simulink model "Noa_Nofusion_backup"  (R2020b)
settings: Solver=FixedStepDiscrete  StartTime=0.0  StopTime=Inf  FixedStep=0.02  RelTol=1e-3
PostLoadFcn:
  | if any(exist('dsrtsu_mdlpostloadfcn', 'file') ~= 0), dsrtsu_mdlpostloadfcn('Execute', bdroot); end
InitFcn:
  | , if any(exist('rtifpga_mdlclblib', 'file') ~= 0), rtifpga_mdlclblib('Init', bdroot); end,
  | , if any(exist('dsmpb_private', 'file') ~= 0), dsmpb_private('dsmpb_mdlclblib', 'Init', bdroot); end,
undefined symbols (not defined in the file): ACC_TimeGap_DecSetSwt, ACC_TimeGap_IncSetSwt, AccelPedalPosn, AccelPedalPosnVldty, AccelPedlPosnDiagc, AccPedalOverride, ACU_ShiftInProgress, ADAS_Posn_CurLane, AESSwtReq, ALC_SwtReq, BrkPedalSts, CC_ACC_CANCEL_OFFSwt, CC_ACC_CRUISE_OFFSwt, CC_ACC_DecSetSpd_SetSwt, CC_ACC_IncSetSpd_ResuSwt, CC_ACCSwtErr, CharSpd_ms, CSA_NODE, CURRENT_GEAR, CurrentGearValid, DiscIntNeverNeededParam, DrvDoorSts, DrvSBR, DrvTrqReqOvld, ECMACCInterface, ECMRespACC, ELKSwtReq, EngLimpHomeSts, EngSpd, EngState, EngState_PHEV, EngTrqMaxActSpd, EngTrqMinAct, EPS_DrvInpTrqVal_HighReslolution, EPS_FailSts, EPS_LKATorqOvrlDlvd, EPS_LKATorqOvrlDlvdVld, EPS_LKATrqOvlDlvdSts, EPS_SteerMod, EPS_TrqSnsrSts, EQ4_APPINFO, EQ4_LA_ELEM, EQ4_LA_HDR, EQ4_LAP_ELEM, EQ4_LAP_HDR, EQ4_LH_ELEM, EQ4_LH_HDR, EQ4_LRE_ELEM, EQ4_LRE_HDR, ESS_PedSwtReq, ESS_VehSwtReq, FFogLmpSts_F_Pbox, FLWheelDriveDirection, FLWheelSpd, FrntWiprSwtSts, FrntWshrSwtSts, FRWheelDriveDirection, FRWheelSpd, HazardLmpSwtSts, HCU_AccelPedalPosn_Diag ... (+152)
libraries: simulink x117, dsmpblib x30
(part 9 of 11)

== system Noa_Nofusion_backup/Common/Subsystem7/DS/DriverStsConditnJudge/DSOther2Hi1DrowsnsJudge ==
  note: %Note
      | Conditions of drowsns state from other state to High 1 as follow:
      | DMSSts_ACC is 0x02: Active
      | && HeadDetn is 0x01: Yes
      | && DrowsnsLevel_ACC is 0x3: Hi level Drowsiness
      | && DrowsnsQlty_ACC≥85%
      | && During time≥0.5s(adjustable)
  canDMSSts : Inport
  canHeadDetn : Inport  Port=2
  canDrowsnsLevel : Inport  Port=3
  PtDSOther2Hi1Drowsns : Inport  Port=4
  Compare To Constant : simulink/Logic and Bit Operations/Compare To Constant  relop===  const=2  OutDataTypeStr=boolean
  Compare To Constant1 : simulink/Logic and Bit Operations/Compare To Constant  relop===  const=1  OutDataTypeStr=boolean
  Compare To Constant2 : simulink/Logic and Bit Operations/Compare To Constant  relop===  const=3  OutDataTypeStr=boolean
  Data Type Conversion : DataTypeConversion  OutDataTypeStr=single
  Logical Operator : Logic  Inputs=3  AllPortsSameDT=off  OutDataTypeStr=boolean
  Relational Operator : RelationalOperator  OutDataTypeStr=boolean  RndMeth=Simplest
  counter : DiscreteIntegrator  ExternalReset=either  SampleTime=-1  LimitOutput=on  UpperSaturationLimit=10  LowerSaturationLimit=-10  ICPrevOutput=DiscIntNeverNeededParam  ICPrevScaledInput=DiscIntNeverNeededParam
  DSOther2Hi1Drowsns : Outport
  wires:
  counter/1 -> Relational Operator/1
  Relational Operator/1 -> DSOther2Hi1Drowsns/1
  Compare To Constant2/1 -> Logical Operator/3
  Compare To Constant/1 -> Logical Operator/1
  Compare To Constant1/1 -> Logical Operator/2
  canDrowsnsLevel/1 -> Compare To Constant2/1
  canHeadDetn/1 -> Compare To Constant1/1
  canDMSSts/1 -> Compare To Constant/1
  Logical Operator/1 -> Data Type Conversion/1
  PtDSOther2Hi1Drowsns/1 -> Relational Operator/2
  Data Type Conversion/1 -> counter/2, counter/1

== system Noa_Nofusion_backup/Common/Subsystem7/DS/DriverStsConditnJudge/DSOther2Hi2DistractnJudge ==
  note: %Note
      | Conditions of distraction state from other state to High 2 as follow:
      | DMSSts_ACC is 0x02: Active
      | && HeadDetn is 0x01: Yes
      | && DistrctnLevel_ACC is 0x03: Hi level distraction
      | && DistrctnQlty_ACC≥ 85%
      | && During time≥5s(adjustable)
  canDMSSts : Inport
  canHeadDetn : Inport  Port=2
  canDistrctnLevel : Inport  Port=3
  canDistrctnQlty : Inport  Port=4
  PtDSOther2Hi2Distractn : Inport  Port=5
  Compare To Constant : simulink/Logic and Bit Operations/Compare To Constant  relop===  const=2  OutDataTypeStr=boolean
  Compare To Constant1 : simulink/Logic and Bit Operations/Compare To Constant  relop===  const=1  OutDataTypeStr=boolean
  Compare To Constant2 : simulink/Logic and Bit Operations/Compare To Constant  relop===  const=3  OutDataTypeStr=boolean
  Compare To Constant4 : simulink/Logic and Bit Operations/Compare To Constant  relop=>=  const=85  OutDataTypeStr=boolean
  Compare To Constant8 : simulink/Logic and Bit Operations/Compare To Constant  relop=<=  const=100  OutDataTypeStr=boolean
  Data Type Conversion : DataTypeConversion  OutDataTypeStr=single
  Logical Operator : Logic  Inputs=5  AllPortsSameDT=off  OutDataTypeStr=boolean
  Relational Operator : RelationalOperator  OutDataTypeStr=boolean  RndMeth=Simplest
  counter : DiscreteIntegrator  ExternalReset=either  SampleTime=-1  LimitOutput=on  UpperSaturationLimit=10  LowerSaturationLimit=-10  ICPrevOutput=DiscIntNeverNeededParam  ICPrevScaledInput=DiscIntNeverNeededParam
  DSOther2Hi2Distractn : Outport
  wires:
  counter/1 -> Relational Operator/1
  Relational Operator/1 -> DSOther2Hi2Distractn/1
  Compare To Constant8/1 -> Logical Operator/5
  Compare To Constant4/1 -> Logical Operator/4
  Compare To Constant2/1 -> Logical Operator/3
  Compare To Constant/1 -> Logical Operator/1
  Compare To Constant1/1 -> Logical Operator/2
  canDistrctnQlty/1 -> Compare To Constant4/1, Compare To Constant8/1
  canDistrctnLevel/1 -> Compare To Constant2/1
  canHeadDetn/1 -> Compare To Constant1/1
  canDMSSts/1 -> Compare To Constant/1
  Logical Operator/1 -> Data Type Conversion/1
  PtDSOther2Hi2Distractn/1 -> Relational Operator/2
  Data Type Conversion/1 -> counter/2, counter/1

== system Noa_Nofusion_backup/Common/Subsystem7/DS/DriverStsConditnJudge/DSOther2Hi2DrowsnsJudge ==
  note: %Note
      | Conditions of drowsns state from other state to High2 as follow:
      | DMSSts_ACC is 0x02: Active
      | && HeadDetn is 0x01: Yes
      | && DrowsnsLevel_ACC is 0x3: Hi level Drowsiness
      | && DrowsnsQlty_ACC≥85%
      | && During time≥3s(adjustable)
  canDMSSts : Inport
  canHeadDetn : Inport  Port=2
  canDrowsnsLevel : Inport  Port=3
  PtDSOther2Hi2Drowsns : Inport  Port=4
  Compare To Constant : simulink/Logic and Bit Operations/Compare To Constant  relop===  const=2  OutDataTypeStr=boolean
  Compare To Constant1 : simulink/Logic and Bit Operations/Compare To Constant  relop===  const=1  OutDataTypeStr=boolean
  Compare To Constant2 : simulink/Logic and Bit Operations/Compare To Constant  relop===  const=3  OutDataTypeStr=boolean
  Data Type Conversion : DataTypeConversion  OutDataTypeStr=single
  Logical Operator : Logic  Inputs=3  AllPortsSameDT=off  OutDataTypeStr=boolean
  Relational Operator : RelationalOperator  OutDataTypeStr=boolean  RndMeth=Simplest
  counter : DiscreteIntegrator  ExternalReset=either  SampleTime=-1  LimitOutput=on  UpperSaturationLimit=10  LowerSaturationLimit=-10  ICPrevOutput=DiscIntNeverNeededParam  ICPrevScaledInput=DiscIntNeverNeededParam
  DSOther2Hi2Drowsns : Outport
  wires:
  Logical Operator/1 -> Data Type Conversion/1
  canDMSSts/1 -> Compare To Constant/1
  canHeadDetn/1 -> Compare To Constant1/1
  canDrowsnsLevel/1 -> Compare To Constant2/1
  Relational Operator/1 -> DSOther2Hi2Drowsns/1
  Compare To Constant1/1 -> Logical Operator/2
  Compare To Constant/1 -> Logical Operator/1
  Compare To Constant2/1 -> Logical Operator/3
  counter/1 -> Relational Operator/1
  PtDSOther2Hi2Drowsns/1 -> Relational Operator/2
  Data Type Conversion/1 -> counter/2, counter/1

== system Noa_Nofusion_backup/Common/Subsystem7/DS/DriverStsConditnJudge/DSOther2UnbelivJudge ==
  note: %Note
      | Conditions of distraction and drowsns state from other to unbelievable as follow:
      | (DMSSts_ACC is no 0x02: Active&& during time ≥3cycles)
      | ∥ (HeadDetn is 0x00: No&&during time≥3s)
      | ∥(DistrctnLevel_ACC is 0x7: Invalid &&during time≥3s)
      | ∥(DrowsnsLevel_ACC is 0x7: Invalid &&during time≥3s)
      | ∥{DistrctnQlty_ACC is 0x7F:Invalid data &&during time≥3s}
      | ∥{DrowsnsQlty_ACC is 0x7F:Invalid data &&during time≥3s}
  canDMSSts : Inport
  canHeadDetn : Inport  Port=2
  canDistrctnLevel : Inport  Port=3
  canDistrctnQlty : Inport  Port=4
  canDrowsnsLevel : Inport  Port=5
  Compare To Constant : simulink/Logic and Bit Operations/Compare To Constant  relop=~=  const=2  OutDataTypeStr=boolean
  Compare To Constant1 : simulink/Logic and Bit Operations/Compare To Constant  relop===  const=0  OutDataTypeStr=boolean
  Compare To Constant{4,9..11} (4 alike) : simulink/Logic and Bit Operations/Compare To Constant  relop=>=  const=3  OutDataTypeStr=boolean
  Compare To Constant2 : simulink/Logic and Bit Operations/Compare To Constant  relop===  const=7  OutDataTypeStr=boolean
  Compare To Constant3 : simulink/Logic and Bit Operations/Compare To Constant  relop===  const=127  OutDataTypeStr=boolean
  Compare To Constant6 : simulink/Logic and Bit Operations/Compare To Constant  relop===  const=7  OutDataTypeStr=boolean
  Data Type Conversion{,1..4} (5 alike) : DataTypeConversion  OutDataTypeStr=single
  Logical Operator : Logic  Operator=OR  Inputs=5  AllPortsSameDT=off  OutDataTypeStr=boolean
  counter{,1..4} (5 alike) : DiscreteIntegrator  ExternalReset=either  SampleTime=-1  LimitOutput=on  UpperSaturationLimit=10  LowerSaturationLimit=-10  ICPrevOutput=DiscIntNeverNeededParam  ICPrevScaledInput=DiscIntNeverNeededParam
  tCycle3plus : simulink/Logic and Bit Operations/Compare To Constant  relop=>=  const=0.06  OutDataTypeStr=boolean
  DSOther2Unbeliv : Outport
  wires:
  Logical Operator/1 -> DSOther2Unbeliv/1
  canDrowsnsLevel/1 -> Compare To Constant6/1
  canDistrctnQlty/1 -> Compare To Constant3/1
  canDistrctnLevel/1 -> Compare To Constant2/1
  canHeadDetn/1 -> Compare To Constant1/1
  canDMSSts/1 -> Compare To Constant/1
  Compare To Constant1/1 -> Data Type Conversion1/1
  Compare To Constant2/1 -> Data Type Conversion2/1
  Compare To Constant6/1 -> Data Type Conversion3/1
  Compare To Constant3/1 -> Data Type Conversion4/1
  Compare To Constant10/1 -> Logical Operator/3
  Compare To Constant11/1 -> Logical Operator/4
  Compare To Constant9/1 -> Logical Operator/2
  Compare To Constant4/1 -> Logical Operator/5
  tCycle3plus/1 -> Logical Operator/1
  Compare To Constant/1 -> Data Type Conversion/1
  counter/1 -> tCycle3plus/1
  counter1/1 -> Compare To Constant9/1
  counter2/1 -> Compare To Constant10/1
  counter3/1 -> Compare To Constant11/1
  counter4/1 -> Compare To Constant4/1
  Data Type Conversion/1 -> counter/2, counter/1
  Data Type Conversion1/1 -> counter1/2, counter1/1
  Data Type Conversion2/1 -> counter2/2, counter2/1
  Data Type Conversion3/1 -> counter3/2, counter3/1
  Data Type Conversion4/1 -> counter4/2, counter4/1

== system Noa_Nofusion_backup/Common/Subsystem7/DS/DriverStsConditnJudge/DSUnbeliv2DDAJudge ==
  note: %Note
      | Following condition aims to prevent transition between DDA and Unbelievable constantly
      | DMSSts_ACC is 0x02: Active&&
      | HeadDetn is 0x01: Yes &&
      | DistrctnLevel_ACC is no 0x7: Invalid&&
      | DrowsnsLevel_ACC is no 0x7: Invalid&&
      | DistrctnQlty_ACC is no 0x7F:Invalid&&
      | DrowsnsQlty_ACC is no 0x7F:Invalid
  canDMSSts : Inport
  canHeadDetn : Inport  Port=2
  canDistrctnLevel : Inport  Port=3
  canDistrctnQlty : Inport  Port=4
  canDrowsnsLevel : Inport  Port=5
  Compare To Constant : simulink/Logic and Bit Operations/Compare To Constant  relop===  const=2  OutDataTypeStr=boolean
  Compare To Constant1 : simulink/Logic and Bit Operations/Compare To Constant  relop===  const=1  OutDataTypeStr=boolean
  Compare To Constant2 : simulink/Logic and Bit Operations/Compare To Constant  relop=~=  const=7  OutDataTypeStr=boolean
  Compare To Constant3 : simulink/Logic and Bit Operations/Compare To Constant  relop=~=  const=127  OutDataTypeStr=boolean
  Compare To Constant6 : simulink/Logic and Bit Operations/Compare To Constant  relop=~=  const=7  OutDataTypeStr=boolean
  Logical Operator : Logic  Inputs=5  AllPortsSameDT=off  OutDataTypeStr=boolean
  DSUnbeliv2DDAEnable : Outport
  wires:
  canDMSSts/1 -> Compare To Constant/1
  canHeadDetn/1 -> Compare To Constant1/1
  canDistrctnLevel/1 -> Compare To Constant2/1
  canDistrctnQlty/1 -> Compare To Constant3/1
  canDrowsnsLevel/1 -> Compare To Constant6/1
  Logical Operator/1 -> DSUnbeliv2DDAEnable/1
  Compare To Constant/1 -> Logical Operator/1
  Compare To Constant1/1 -> Logical Operator/2
  Compare To Constant2/1 -> Logical Operator/3
  Compare To Constant6/1 -> Logical Operator/4
  Compare To Constant3/1 -> Logical Operator/5

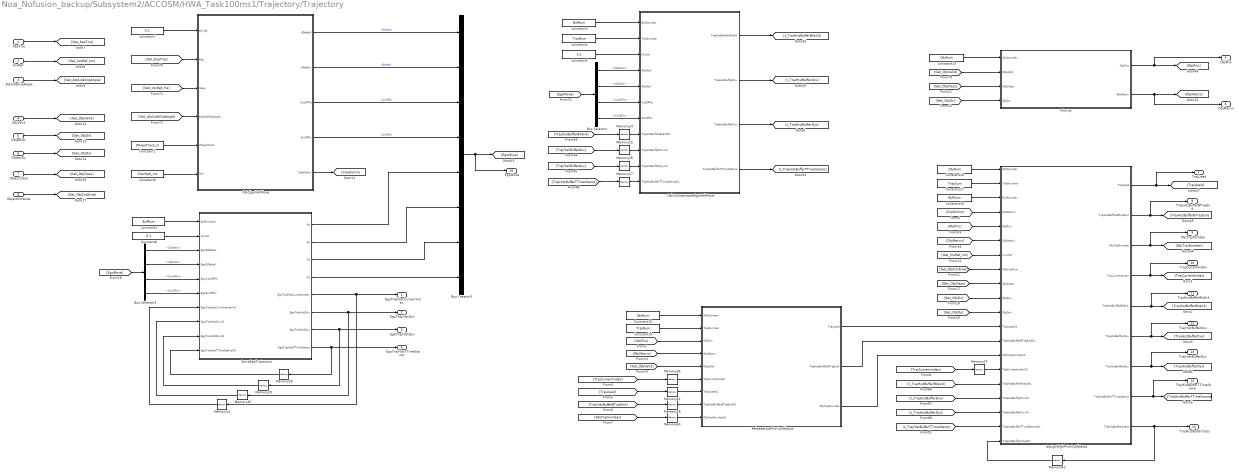
== system Noa_Nofusion_backup/Subsystem2/ACCOSM/HWA_Task100ms1/Trajectory/Trajectory ==
  KapTraj : Inport
  VxvRef : Inport  Port=2
  AlpSideSlipAngle : Inport  Port=3
  ObjValid : Inport  Port=4
  ObjectDx : Inport  Port=5
  ObjectDy : Inport  Port=6
  ObjectClass : Inport  Port=7
  ObjectCntAlive : Inport  Port=8
  AssignHighPriorityObjects : MATLAB Function  TreatAsAtomicUnit=on
  Bus Creator3 : BusCreator  Inputs=8
  Bus Selector : BusSelector  OutputSignals=dDeltaX,dDeltaY,CosOfPsi,SinOfPsi
  Bus Selector3 : BusSelector  OutputSignals=dDeltaX,dDeltaY,CosOfPsi,SinOfPsi
  CalcCompensateEgoVehMove : MATLAB Function  TreatAsAtomicUnit=on
  CalcEgoVehMove : MATLAB Function  TreatAsAtomicUnit=on
  Constant1 : Constant  Value=WheelTrack_m  OutDataTypeStr=single
  Constant13 : Constant  Value=ObjNum  OutDataTypeStr=uint8
  Constant14 : Constant  Value=TrajNum  OutDataTypeStr=uint8
  Constant15 : Constant  Value=ObjNum  OutDataTypeStr=uint8
  Constant16 : Constant  Value=BufNum  OutDataTypeStr=uint8
  Constant17 : Constant  Value=TrajNum  OutDataTypeStr=uint8
  Constant18 : Constant  Value=ObjNum  OutDataTypeStr=uint8
  Constant2 : Constant  Value=BufNum  OutDataTypeStr=uint8
  Constant3 : Constant  Value=BufNum  OutDataTypeStr=uint8
  Constant4 : Constant  Value=TrajNum  OutDataTypeStr=uint8
  Constant5 : Constant  Value=0.1  OutDataTypeStr=single
  Constant6 : Constant  Value=0.1  OutDataTypeStr=single
  Constant7 : Constant  Value=0.1  OutDataTypeStr=single
  Constant8 : Constant  Value=CharSpd_ms  OutDataTypeStr=single
  Memory{24..26,42} (4 alike) : Memory  InitialCondition=zeros(TrajNum,BufNum)  InheritSampleTime=on
  Memory27 : Memory  InitialCondition=32*ones(TrajNum,BufNum)  InheritSampleTime=on
  Memory28 : Memory  InitialCondition=32*ones(BufNum,1)  InheritSampleTime=on
  Memory29 : Memory  InitialCondition=zeros(BufNum,1)  InheritSampleTime=on
  Memory30 : Memory  InitialCondition=zeros(BufNum,1)  InheritSampleTime=on
  Memory31 : Memory  InitialCondition=1  InheritSampleTime=on
  Memory36 : Memory  InitialCondition=ones(TrajNum,1)  InheritSampleTime=on
  Memory37 : Memory  InitialCondition=ones(TrajNum,1)  InheritSampleTime=on
  Memory38 : Memory  InitialCondition=ones(TrajNum,BufNum)  InheritSampleTime=on
  Memory40 : Memory  InitialCondition=255*ones(ObjNum,1)  InheritSampleTime=on
  Memory41 : Memory  InitialCondition=zeros(TrajNum,1)  InheritSampleTime=on
  Priority : MATLAB Function  TreatAsAtomicUnit=on
  ReleaseLowPriorityObjects : MATLAB Function  TreatAsAtomicUnit=on
  StoreEgoTrajectory : MATLAB Function  TreatAsAtomicUnit=on
  EgoTrajHistCurrentIndex : Outport
  EgoTrajHistDxv : Outport  Port=2
  EgoTrajHistDyv : Outport  Port=3
  EgoTrajHistTTimeStamp : Outport  Port=4
  ObjPrio : Outport  Port=5
  ObjMatrix : Outport  Port=6
  TrajUsed : Outport  Port=7
  TrajHistBufferBTrajEnd : Outport  Port=8
  ObjTrajNumber : Outport  Port=9
  TrajCurrentIndex : Outport  Port=10
  TrajHistBufferBValid : Outport  Port=11
  TrajHistBufferDxv : Outport  Port=12
  TrajHistBufferDyv : Outport  Port=13
  TrajHistBufferTTimeStamp : Outport  Port=14
  TrajHistBufferClass : Outport  Port=15
  EgoMove : Outport  Port=16
  wires:
  StoreEgoTrajectory/1(Pa) -> Bus Creator3/5
  StoreEgoTrajectory/2(Pb) -> Bus Creator3/6
  StoreEgoTrajectory/3(Pc) -> Bus Creator3/7
  StoreEgoTrajectory/4(Pd) -> Bus Creator3/8
  Bus Creator3/1 -> [EgoMove], EgoMove/1
  [SlipDislim] -> AssignHighPriorityObjects/4(SlipDisLim)
  CalcEgoVehMove/5(SlipDislim) -> [SlipDislim]
  Constant8/1 -> CalcEgoVehMove/6(Vch)
  Constant1/1 -> CalcEgoVehMove/5(WheelTrack)
  CalcCompensateEgoVehMove/3(TrajHistBufferDyv) -> [t_TrajHistBufferDyv]
  Priority/2(ObjMatrix) -> ObjMatrix/1, [ObjMatrix]
  Priority/1(ObjPrio) -> [ObjPrio], ObjPrio/1
  CalcEgoVehMove/4(SinOfPsi) -> Bus Creator3/4  "SinOfPsi"
  CalcEgoVehMove/3(CosOfPsi) -> Bus Creator3/3  "CosOfPsi"
  CalcEgoVehMove/2(dDeltaY) -> Bus Creator3/2  "dDeltaY"
  CalcEgoVehMove/1(dDeltaX) -> Bus Creator3/1  "dDeltaX"
  ObjectCntAlive/1 -> [Get_ObjCntAlive]
  ObjectClass/1 -> [Get_ObjClass]
  ObjectDx/1 -> [Get_ObjDx]
  ObjectDy/1 -> [Get_ObjDy]
  ObjValid/1 -> [Get_ObjValid]
  AssignHighPriorityObjects/8(TrajHistBufferTTimeStamp) -> [TrajHistBufferTTimeStamp], TrajHistBufferTTimeStamp/1
  Bus Selector3/1 -> StoreEgoTrajectory/3(EgoDDeltaX)  "<dDeltaX>"
  Bus Selector3/4 -> StoreEgoTrajectory/6(EgoSinOfPsi)  "<SinOfPsi>"
  Bus Selector3/2 -> StoreEgoTrajectory/4(EgoDDeltaY)  "<dDeltaY>"
  Bus Selector3/3 -> StoreEgoTrajectory/5(EgoCosOfPsi)  "<CosOfPsi>"
  StoreEgoTrajectory/8(EgoTrajHistTTimeStamp) -> Memory28/1, EgoTrajHistTTimeStamp/1
  Memory31/1 -> StoreEgoTrajectory/7(EgoTrajHistCurrentIndexK1)
  StoreEgoTrajectory/5(EgoTrajHistCurrentIndex) -> Memory31/1, EgoTrajHistCurrentIndex/1
  Memory30/1 -> StoreEgoTrajectory/8(EgoTrajHistDxvK1)
  StoreEgoTrajectory/6(EgoTrajHistDxv) -> Memory30/1, EgoTrajHistDxv/1
  Memory29/1 -> StoreEgoTrajectory/9(EgoTrajHistDyvK1)
  Memory28/1 -> StoreEgoTrajectory/10(EgoTrajHistTTimeStampK1)
  StoreEgoTrajectory/7(EgoTrajHistDyv) -> Memory29/1, EgoTrajHistDyv/1
  Constant6/1 -> StoreEgoTrajectory/2(tCycle)
  Constant2/1 -> StoreEgoTrajectory/1(BufNumber)
  [ObjMatrix] -> AssignHighPriorityObjects/6(ObjMatrix)
  [ObjMatrix] -> ReleaseLowPriorityObjects/4(ObjMatrix)
  Constant16/1 -> AssignHighPriorityObjects/3(BufNumber)
  Constant17/1 -> AssignHighPriorityObjects/2(TrajNumber)
  Constant18/1 -> AssignHighPriorityObjects/1(ObjNumber)
  Constant14/1 -> ReleaseLowPriorityObjects/2(TrajNumber)
  Constant15/1 -> ReleaseLowPriorityObjects/1(ObjNumber)
  Constant13/1 -> Priority/1(ObjNumber)
  Constant4/1 -> CalcCompensateEgoVehMove/2(TrajNumber)
  Constant3/1 -> CalcCompensateEgoVehMove/1(BufNumber)
  AlpSideSlipAngle/1 -> [Get_AlpSideSlipAngle]
  VxvRef/1 -> [Get_VxvRef_ms]
  KapTraj/1 -> [Get_KapTraj]
  [Get_ObjCntAlive] -> AssignHighPriorityObjects/8(ObjCntAlive)
  [TrajHistBufferBValid] -> Memory24/1
  [TrajHistBufferDyv] -> Memory26/1
  [TrajHistBufferDxv] -> Memory25/1
  [TrajHistBufferTTimeStamp] -> Memory27/1
  [Get_ObjDy] -> AssignHighPriorityObjects/11(ObjDyv)
  AssignHighPriorityObjects/4(TrajCurrentIndex) -> [TrajCurrentIndex], TrajCurrentIndex/1
  [Get_ObjDx] -> AssignHighPriorityObjects/10(ObjDxv)
  [Get_ObjClass] -> AssignHighPriorityObjects/9(ObjClass)
  [Get_VxvRef_ms] -> AssignHighPriorityObjects/7(VxvRef)
  [TrajCurrentIndex] -> Memory37/1
  [TrajCurrentIndex] -> Memory36/1
  AssignHighPriorityObjects/6(TrajHistBufferDxv) -> [TrajHistBufferDxv], TrajHistBufferDxv/1
  AssignHighPriorityObjects/7(TrajHistBufferDyv) -> [TrajHistBufferDyv], TrajHistBufferDyv/1
  AssignHighPriorityObjects/5(TrajHistBufferBValid) -> [TrajHistBufferBValid], TrajHistBufferBValid/1
  [Get_ObjValid] -> ReleaseLowPriorityObjects/5(ObjValid)
  [ObjPrio] -> ReleaseLowPriorityObjects/3(ObjPrio)
  [TrajHistBufferBTrajEnd] -> Memory38/1
  [ObjTrajNumber] -> Memory40/1
  [TrajUsed] -> Memory41/1
  Memory42/1 -> AssignHighPriorityObjects/20(TrajHistBufferClassK1)
  Memory41/1 -> ReleaseLowPriorityObjects/7(TrajUsedK1)
  Memory40/1 -> ReleaseLowPriorityObjects/9(ObjTrajNumberK1)
  Memory38/1 -> ReleaseLowPriorityObjects/8(TrajHistBufferBTrajEndK1)
  Memory37/1 -> AssignHighPriorityObjects/15(TrajCurrentIndexK1)
  Memory36/1 -> ReleaseLowPriorityObjects/6(TrajCurrentIndex)
  [t_TrajHistBufferTTimeStamp] -> AssignHighPriorityObjects/19(TrajHistBufferTTimeStampK1)
  CalcCompensateEgoVehMove/4(TrajHistBufferTTimeStamp) -> [t_TrajHistBufferTTimeStamp]
  [t_TrajHistBufferDyv] -> AssignHighPriorityObjects/18(TrajHistBufferDyvK1)
  [t_TrajHistBufferDxv] -> AssignHighPriorityObjects/17(TrajHistBufferDxvK1)
  CalcCompensateEgoVehMove/2(TrajHistBufferDxv) -> [t_TrajHistBufferDxv]
  [t_TrajHistBufferBValid] -> AssignHighPriorityObjects/16(TrajHistBufferBValidK1)
  CalcCompensateEgoVehMove/1(TrajHistBufferBValid) -> [t_TrajHistBufferBValid]
  [ObjPrio] -> AssignHighPriorityObjects/5(ObjPrio)
  AssignHighPriorityObjects/9(TrajHistBufferClass) -> TrajHistBufferClass/1, Memory42/1
  AssignHighPriorityObjects/2(TrajHistBufferBTrajEnd) -> [TrajHistBufferBTrajEnd], TrajHistBufferBTrajEnd/1
  AssignHighPriorityObjects/1(TrajUsed) -> [TrajUsed], TrajUsed/1
  ReleaseLowPriorityObjects/3(ObjTrajNumber) -> AssignHighPriorityObjects/14(ObjTrajNumberK1)
  AssignHighPriorityObjects/3(ObjTrajNumber) -> [ObjTrajNumber], ObjTrajNumber/1
  ReleaseLowPriorityObjects/1(TrajUsed) -> AssignHighPriorityObjects/12(TrajUsedK1)
  ReleaseLowPriorityObjects/2(TrajHistBufferBTrajEnd) -> AssignHighPriorityObjects/13(TrajHistBufferBTrajEndK1)
  [Get_ObjValid] -> Priority/2(ObjValid)
  [Get_ObjClass] -> Priority/3(ObjClass)
  [Get_ObjDx] -> Priority/4(ObjDx)
  [EgoMove] -> Bus Selector3/1
  Bus Selector/4 -> CalcCompensateEgoVehMove/7(SinOfPsi)  "<SinOfPsi>"
  Bus Selector/3 -> CalcCompensateEgoVehMove/6(CosOfPsi)  "<CosOfPsi>"
  Bus Selector/2 -> CalcCompensateEgoVehMove/5(dDeltaY)  "<dDeltaY>"
  Bus Selector/1 -> CalcCompensateEgoVehMove/4(dDeltaX)  "<dDeltaX>"
  [EgoMove] -> Bus Selector/1
  Memory27/1 -> CalcCompensateEgoVehMove/11(TrajHistBufferTTimeStampK1)
  Memory26/1 -> CalcCompensateEgoVehMove/10(TrajHistBufferDyvK1)
  Memory25/1 -> CalcCompensateEgoVehMove/9(TrajHistBufferDxvK1)
  Memory24/1 -> CalcCompensateEgoVehMove/8(TrajHistBufferBValidK1)
  Constant5/1 -> CalcCompensateEgoVehMove/3(tCycle)
  [Get_KapTraj] -> CalcEgoVehMove/2(Kap)
  [Get_AlpSideSlipAngle] -> CalcEgoVehMove/4(alpSideSlipAngle)
  [Get_VxvRef_ms] -> CalcEgoVehMove/3(Vego)
  Constant7/1 -> CalcEgoVehMove/1(tCycle)

== system Noa_Nofusion_backup/Subsystem2/ACCOSM/ObjMatrixTransit/Subsystem/For Each Subsystem ==
  <EQ4_OBJ_ELEM> : Inport  Partition=on  PartitionDimension=1  PartitionWidth=1  PartitionOffset=0
  Bus Selector : BusSelector  OutputSignals=OBJ_ID,OBJ_Existence_Probability,OBJ_Object_Class,OBJ_Width,OBJ_Long_Distance,OBJ_Lat_Distance,OBJ_Abs_Long_Acc,OBJ_Abs_Long_Velocity,OBJ_Abs_Lat_Velocity,OBJ_Brake_Light,OBJ_Object_Age,OBJ_Motion_Status,OBJ_Motion_Category,OBJ_Motion_Orientation
  For Each : ForEach  DisableCoverage=on
  id : Outport  ConcatenationDimension=1
  confidence : Outport  Port=2  ConcatenationDimension=1
  classification : Outport  Port=3  ConcatenationDimension=1
  width : Outport  Port=4  ConcatenationDimension=1
  LongDis : Outport  Port=5  ConcatenationDimension=1
  LatDis : Outport  Port=6  ConcatenationDimension=1
  AbsLongAcc : Outport  Port=7  ConcatenationDimension=1
  AbsLongVel : Outport  Port=8  ConcatenationDimension=1
  AbsLatVel : Outport  Port=9  ConcatenationDimension=1
  BrakeLight : Outport  Port=10  ConcatenationDimension=1
  Age : Outport  Port=11  ConcatenationDimension=1
  motionSts : Outport  Port=12  ConcatenationDimension=1
  motionCategory : Outport  Port=13  ConcatenationDimension=1
  motionOrientation : Outport  Port=14  ConcatenationDimension=1
  wires:
  Bus Selector/13 -> motionCategory/1  "<OBJ_Motion_Category>"
  Bus Selector/3 -> classification/1  "<OBJ_Object_Class>"
  Bus Selector/14 -> motionOrientation/1  "<OBJ_Motion_Orientation>"
  Bus Selector/4 -> width/1  "<OBJ_Width>"
  Bus Selector/11 -> Age/1  "<OBJ_Object_Age>"
  Bus Selector/5 -> LongDis/1  "<OBJ_Long_Distance>"
  Bus Selector/8 -> AbsLongVel/1  "<OBJ_Abs_Long_Velocity>"
  Bus Selector/10 -> BrakeLight/1  "<OBJ_Brake_Light>"
  Bus Selector/2 -> confidence/1  "<OBJ_Existence_Probability>"
  Bus Selector/1 -> id/1  "<OBJ_ID>"
  Bus Selector/7 -> AbsLongAcc/1  "<OBJ_Abs_Long_Acc>"
  Bus Selector/9 -> AbsLatVel/1  "<OBJ_Abs_Lat_Velocity>"
  Bus Selector/6 -> LatDis/1  "<OBJ_Lat_Distance>"
  Bus Selector/12 -> motionSts/1  "<OBJ_Motion_Status>"
  <EQ4_OBJ_ELEM>/1 -> Bus Selector/1

== system Noa_Nofusion_backup/Subsystem2/ACCOSM/ObjMatrixTransit/Subsystem/For Iterator Subsystem ==
  <EQ4_OBJ_ELEM> : Inport
  Bus Selector : BusSelector  OutputSignals=OBJ_ID,OBJ_Existence_Probability,OBJ_Object_Class,OBJ_Width,OBJ_Long_Distance,OBJ_Lat_Distance,OBJ_Abs_Long_Acc,OBJ_Abs_Long_Velocity,OBJ_Abs_Lat_Velocity,OBJ_Brake_Light,OBJ_Object_Age,OBJ_Motion_Status,OBJ_Motion_Category,OBJ_Motion_Orientation
  For Iterator : ForIterator  IterationLimit=20
  Selector : Selector  InputPortWidth=20  IndexOptions=Index vector (port)  Indices=[1 3]  OutputSizes=1
  id : Outport
  confidence : Outport  Port=2
  classification : Outport  Port=3
  width : Outport  Port=4
  LongDis : Outport  Port=5
  LatDis : Outport  Port=6
  AbsLongAcc : Outport  Port=7
  AbsLongVel : Outport  Port=8
  AbsLatVel : Outport  Port=9
  BrakeLight : Outport  Port=10
  Age : Outport  Port=11
  motionSts : Outport  Port=12
  motionCategory : Outport  Port=13
  motionOrientation : Outport  Port=14
  wires:
  Bus Selector/14 -> motionOrientation/1  "<OBJ_Motion_Orientation>"
  Bus Selector/13 -> motionCategory/1  "<OBJ_Motion_Category>"
  Bus Selector/12 -> motionSts/1  "<OBJ_Motion_Status>"
  Bus Selector/11 -> Age/1  "<OBJ_Object_Age>"
  Bus Selector/10 -> BrakeLight/1  "<OBJ_Brake_Light>"
  Bus Selector/9 -> AbsLatVel/1  "<OBJ_Abs_Lat_Velocity>"
  Bus Selector/8 -> AbsLongVel/1  "<OBJ_Abs_Long_Velocity>"
  Bus Selector/7 -> AbsLongAcc/1  "<OBJ_Abs_Long_Acc>"
  Bus Selector/6 -> LatDis/1  "<OBJ_Lat_Distance>"
  Bus Selector/5 -> LongDis/1  "<OBJ_Long_Distance>"
  Bus Selector/4 -> width/1  "<OBJ_Width>"
  Bus Selector/3 -> classification/1  "<OBJ_Object_Class>"
  Bus Selector/2 -> confidence/1  "<OBJ_Existence_Probability>"
  Bus Selector/1 -> id/1  "<OBJ_ID>"
  Selector/1 -> Bus Selector/1
  For Iterator/1 -> Selector/2
  <EQ4_OBJ_ELEM>/1 -> Selector/1

== matlab function Noa_Nofusion_backup/Subsystem2/ACCOSM/HWA_Task100ms1/Lpb ==
  data: vRef input single size=1; alpSumSlideCurveness input single size=1; ObjValid input boolean size=15; ObjDyc input single size=15; ObjLpb output single size=15; ObjDycHist input single size=15; ObjqDycHist input single size=15; ObjLpbL output single size=15; ObjLpbR output single size=15; ObjVyc input single size=15; ObjYawAngle input single size=15; ObjDylaneEdgeRight input; ObjDyEdgeWidthRight input; ObjDylaneEdgeLeft input; ObjDyEdgeWidthLeft input
function [ObjLpb,ObjLpbL,ObjLpbR] = LpbCalc(vRef,alpSumSlideCurveness,...
    ObjValid,ObjDyc,ObjDycHist,ObjqDycHist,ObjVyc,ObjYawAngle,...
    ObjDylaneEdgeRight,ObjDyEdgeWidthRight,ObjDylaneEdgeLeft,ObjDyEdgeWidthLeft)

 [ObjLpb,ObjLpbL,ObjLpbR] = LpbCalc(vRef,alpSumSlideCurveness,...
    ObjValid,ObjDyc,ObjDycHist,ObjqDycHist,ObjVyc,ObjYawAngle,...
    ObjDylaneEdgeRight,ObjDyEdgeWidthRight,ObjDylaneEdgeLeft,ObjDyEdgeWidthLeft);
end

== matlab function Noa_Nofusion_backup/Subsystem2/ACCOSM/HWA_Task100ms1/Plaus ==
  data: dxMaxFollow input single size=1; ObjValid input boolean size=15; ObjDx input single size=15; ObjVx input single size=15; ObjPlaus output single size=15; ObjOnLeft input single size=15; ObjPlausLeft output single size=15; ObjPlausRight output single size=15; ObjOnRight input single size=15; ObjDycHist input single size=15; ObjqDycHist input single size=15; ObjLpb input single size=15; ObjLpbLeft input single size=15; ObjLpbRight input single size=15; ObjPlausK1 input single size=15; ObjPlausLeftK1 input single size=15; ObjPlausRightK1 input single size=15
function [ObjPlaus,ObjPlausLeft,ObjPlausRight] = ...
    PlausCalc(dxMaxFollow,ObjValid,ObjDx,ObjVx,ObjOnLeft,ObjOnRight,ObjDycHist,ObjqDycHist,...
    ObjLpb,ObjLpbLeft,ObjLpbRight,ObjPlausK1,ObjPlausLeftK1,ObjPlausRightK1)

[ObjPlaus,ObjPlausLeft,ObjPlausRight] = ...
    PlausCalc(dxMaxFollow,ObjValid,ObjDx,ObjVx,ObjOnLeft,ObjOnRight,ObjDycHist,ObjqDycHist,...
    ObjLpb,ObjLpbLeft,ObjLpbRight,ObjPlausK1,ObjPlausLeftK1,ObjPlausRightK1);
end

== matlab function Noa_Nofusion_backup/Subsystem2/ACCOSM/HWA_Task100ms1/Spw ==
  data: AlpSumSlideCurveness input single size=1; kapCourseErr input single size=1; ObjSpw output single size=15; ObjValid input boolean size=15; DycASI input single size=15; ObjDx input single size=15; ObjSpwLeft output single size=15; ObjSpwRight output single size=15; ObjOnLeft output; ObjOnRight output; ObjDyc input; ObjDycHist input; ObjqDycHist input; ObjDycASI output; ObjDyKapErr output
function [ObjSpw,ObjSpwLeft,ObjSpwRight,ObjOnLeft,ObjOnRight,ObjDycASI,ObjDyKapErr] = ...
    CalcSpw(AlpSumSlideCurveness,kapCourseErr,ObjValid,DycASI,ObjDx,ObjDyc,ObjDycHist,ObjqDycHist)
 
ObjSpw = single(zeros(15,1));
ObjSpwLeft = single(zeros(15,1));
ObjSpwRight = single(zeros(15,1));
ObjOnLeft = single(zeros(15,1));
ObjOnRight = single(zeros(15,1));
ObjDycASI = single(zeros(15,1));
ObjDyKapErr = single(zeros(15,1));
 
for i=1:15
    if ObjValid(i)
        t_dycASI = DycASI(i);
        t_kapErrMin = single(0.0002);
        t_kapErrCurvenessMax = single(0.0018);
        
        temp1 = min(AlpSumSlideCurveness,single(1));
        t_kapErrCurveness = t_kapErrCurvenessMax*temp1;
        t_kapErr = max(t_kapErrMin,max(kapCourseErr,t_kapErrCurveness));
        temp1 = min(ObjDx(i),single(80));
        t_DyKapErr = t_kapErr*temp1*temp1/2;
        ObjDyKapErr(i) = t_DyKapErr;
        
        %         t_dyHalfLane = 1.5;
        %         t_dy3halfLane = 5.25;
        
        if abs(t_dycASI)>=4.5
            t_spw = single(0);
            t_spwNeighbour = single(0);
        elseif abs(t_dycASI)>=3
            t_spw = single(0);
            t_dycToLane = abs(t_dycASI) - single(3);
            t_spwNeighbour = CalcSPW(t_dycToLane,single(3),t_DyKapErr);
        elseif abs(t_dycASI)>=1.5
            t_spw = single(0);
            t_spwNeighbour = CalcSPW(single(0),single(3),t_DyKapErr);
        else
            t_spwNeighbour = single(0);
            t_spw = CalcSPW(single(0),single(3),t_DyKapErr);
        end
        if t_dycASI>=0
            t_spwRight = single(0);
            t_spwLeft = t_spwNeighbour;
        else
            t_spwLeft = single(0);
            t_spwRight = t_spwNeighbour;
        end
        ObjSpw(i) = t_spw;
        ObjSpwLeft(i) = t_spwLeft;
        ObjSpwRight(i) = t_spwRight;
        % -------------------------------------------------------------------------
        
        temp1 = 0.5*ObjqDycHist(i);
        t_dycASI = ObjDyc(i)*(1-temp1) + ObjDycHist(i)*temp1;
        temp2 = single(1.5) + t_DyKapErr;
        temp3 = single(3) + t_DyKapErr;
        ObjDycASI(i) = t_dycASI;
        
        if t_dycASI>=0
            temp1 = max(single(1.5),min(temp3,t_dycASI)) - single(1.5);
            ObjOnLeft(i) = min(single(1),temp1/temp2);
        else
            temp1 = max(min(single(-1.5),t_dycASI),-temp3);
            temp1 = -temp1 - single(1.5);
            ObjOnRight(i) = min(single(1),temp1/temp2);
        end
    end
end
end
 
function t_spw = CalcSPW(absDyc,dyLaneWidth,dyKapErr)
temp3 = dyLaneWidth/2;
temp1 = temp3 - dyKapErr;
temp2 = temp3 + dyKapErr;
temp2 = min(temp2,dyLaneWidth);
 
if absDyc<=temp1
    t_spw = single(1);
elseif absDyc>=temp2
    t_spw = single(0);
else
    temp3 = temp2 - absDyc;
    temp4 = 2*dyKapErr;
    t_spw = temp3/temp4;
end
end

== matlab function Noa_Nofusion_backup/Subsystem2/ACCOSM/HWA_Task100ms1/Std ==
  data: u input; y output
function y = fcn(u)

y = std(u);

== matlab function Noa_Nofusion_backup/Subsystem2/ACCOSM/HWA_Task100ms1/TargetBrake ==
  data: ID input uint8; VxG input; VyG input; TargetBrake_b output boolean; TargetVxG output; BrakeLightIndic input uint8 size=15; TargetVyG output
function [TargetBrake_b,TargetVxG,TargetVyG] = fcn(ID,VxG,VyG,BrakeLightIndic)
%#codegen
TargetBrake_b = false;
TargetVxG = single(0);
TargetVyG = single(0);

if (ID>0)&&(ID<100)
    if BrakeLightIndic(ID)==2
        TargetBrake_b = true;
    end
    TargetVxG = VxG(ID);
    TargetVyG = VyG(ID);
end

== matlab function Noa_Nofusion_backup/Subsystem2/ACCOSM/HWA_Task100ms1/TargetSelect ==
  data: ACCmode input uint8 size=1; P0ID output uint8 size=1; vRef input single size=1; Valid input boolean size=15; Range input single size=15; Vr input single size=15; Dx input single size=15; Dy input single size=15; ArG input single size=15; Dyc input single size=15; Vyc input single size=15; Cnt input; plaus input single size=15; wCutIn input single size=15; spw input single size=15; spwLeft input single size=15; spwRight input single size=15; ReID input uint8 size=1; ReRange input single size=1; ReArG input single size=1; ReDx input single size=1; ReDy input single size=1; ReVx input single size=1; ReCutIn_b input boolean size=1; ReDyc input single size=1; ReVyc input single size=1; TargetLost_b input; tTargetLost input single size=1; dyLaneWidth input single size=1; Classfication input uint8 size=15; MoveSts input uint8 size=15; TarLimDx input single size=1; TarLimS0Dx input; TargetExistK1 input boolean size=1; P2ID output uint8 size=1; P3ID output uint8 size=1; P0Range output single size=1; P2Range output single size=1; P3Range output single size=1; P0Vr output single size=1; P2Vr output single size=1; P3Vr output single size=1; P0ArG output single size=1; P2ArG output single size=1; P3ArG output single size=1; P0Dx output single size=1; P2Dx output single size=1; P3Dx output single size=1; P0Dy output single size=1; P2Dy output single size=1; P3Dy output single size=1; TargetCutIn_b output boolean size=1; P0Dyc output single size=1; P0Vyc output single size=1; TargetExist output boolean size=1; TargetReplacedCntK1 input uint8; TargetReplacedCnt output uint8
function [P0ID,P2ID,P3ID,P0Range,P2Range,P3Range,P0Vr,P2Vr,P3Vr,P0ArG,P2ArG,P3ArG,...
    P0Dx,P2Dx,P3Dx,P0Dy,P2Dy,P3Dy,TargetCutIn_b,P0Dyc,P0Vyc,TargetExist,TargetReplacedCnt] = ...
    ATS(ACCmode,vRef,Valid,Range,Vr,Dx,Dy,ArG,Dyc,Vyc,Cnt,plaus,wCutIn,spw,spwLeft,spwRight,...
    ReID,ReRange,ReArG,ReDx,ReDy,ReVx,ReCutIn_b,ReDyc,ReVyc,TargetLost_b,tTargetLost,dyLaneWidth,...
    Classfication,MoveSts,TarLimDx,TarLimS0Dx,TargetExistK1,TargetReplacedCntK1)

% #codegen
% ACCMode
% 0x00:OFF mode
% 0x01:Passive mode(Reject)
% 0x02:Passive mode(Stand-by)
% 0x03:Active-Control mode
% 0x04:Brake-only mode
% 0x05:Override
% 0x06:Standstill
% 0x07:Failure mode
% 0x08~0x1F:Reserved

P0ID = uint8(0);
P2ID = uint8(0);
P3ID = uint8(0);
P0Range = single(255);
P2Range = single(255);
P3Range = single(255);
P0Vr = single(0);
P2Vr = single(0);
P3Vr = single(0);
P0ArG = single(0);
P2ArG = single(0);
P3ArG = single(0);
P0Dx = single(255);
P2Dx = single(255);
P3Dx = single(255);
P0Dy = single(0);
P2Dy = single(0);
P3Dy = single(0);
TargetExist = false;
TargetCutIn_b = false;
P0Dyc = single(0);
P0Vyc = single(0);

DycOffset = interpolate(single(50),single(0.35),single(80),single(0.6),ReDx);

if TargetLost_b
   TargetReplacedCnt = uint8(0);
else
   TargetReplacedCnt = min(uint8(255),TargetReplacedCntK1 + uint8(1));
end

if (ACCmode==1)||(ACCmode==2)||(ACCmode==3)||(ACCmode==4)||(ACCmode==5)||(ACCmode==6)||(ACCmode==9)
    if TargetExistK1==false   % first select target
        for i=1:15
            if (Valid(i)==1)&&(Cnt(i)>=3)&&...
                    (((vRef<=15.83)&&((MoveSts(i)==1)||(MoveSts(i)==2)||(MoveSts(i)==3)))||...
                    ((vRef>15.83)&&((MoveSts(i)==2)||(MoveSts(i)==3))))
                if (Classfication(i)==1)||(Classfication(i)==2)||(Classfication(i)==3)||(Classfication(i)==9)
                    if ((Range(i)<=TarLimS0Dx)&&(MoveSts(i)==1))||((Range(i)<=TarLimDx)&&((MoveSts(i)==2)||(MoveSts(i)==3)))
                        if (plaus(i)>=0.4)||((wCutIn(i)>0.7)&&(spw(i)>=0.8))||((spw(i)>0.95)&&(Range(i)<1.5*vRef))         % Need Check!
                            if Range(i)<P0Range
                                P0ID = uint8(i);
                                P0Range = Range(i);
                            end
                        else
                            if spwLeft(i)>0.2
                                if Range(i)<P2Range
                                    P2ID = uint8(i);
                                    P2Range = Range(i);
                                end
                            end
                            if spwRight(i)>0.2
                                if Range(i)<P3Range
                                    P3ID = uint8(i);
                                    P3Range = Range(i);
                                end
                            end
                        end
                    end
                end
            end
        end
    else
        k = ReID;
        if k<100        % No Target Lost!!!
            if (Valid(k)==0)
                for i=1:15
                    if (Valid(i)==1)&&...
                            (((vRef<=15.83)&&((MoveSts(i)==1)||(MoveSts(i)==2)||(MoveSts(i)==3)))||...
                            ((vRef>15.83)&&((MoveSts(i)==2)||(MoveSts(i)==3))))
                        if (Classfication(i)==1)||(Classfication(i)==2)||(Classfication(i)==3)||(Classfication(i)==9)
                            if ((Range(i)<=TarLimS0Dx)&&(MoveSts(i)==1))||((Range(i)<=TarLimDx)&&((MoveSts(i)==2)||(MoveSts(i)==3)))
                                if (plaus(i)>=0.4)||((wCutIn(i)>0.7)&&(spw(i)>=0.8))||((spw(i)>0.95)&&(Range(i)<1.5*vRef))
                                    if Range(i)<P0Range
                                        P0ID = uint8(i);
                                        P0Range = Range(i);
                                    end
                                else
                                    if spwLeft(i)>0.2
                                        if Range(i)<P2Range
                                            P2ID = uint8(i);
                                            P2Range = Range(i);
                                        end
                                    end
                                    if spwRight(i)>0.2
                                        if Range(i)<P3Range
                                            P3ID = uint8(i);
                                            P3Range = Range(i);
                                        end
                                    end
                                end
                            end
                        end
                    end
                end
            else
                temp = interpolate(single(5),single(10),single(30),single(20),vRef);
                
                if TargetReplacedCnt>4   % no Target lost  Or  After Target 4  cnt!
                    if ((Range(k)<=(TarLimS0Dx+temp))&&(MoveSts(k)==1))||((Range(k)<=(TarLimDx+temp))&&((MoveSts(k)==2)||(MoveSts(k)==3)))
                        if (plaus(k)>=0.2)||((wCutIn(k)>0.6)&&(spw(k)>=0.4))||(spw(k)>0.6)
                            if Range(k)<P0Range
                                P0ID = uint8(k);
                                P0Range = Range(k);
                            end
                        else
                            if spwLeft(k)>0.2
                                if Range(k)<P2Range
                                    P2ID = uint8(k);
                                    P2Range = Range(k);
                                end
                            end
                            if spwLeft(k)>0.2
                                if Range(k)<P3Range
                                    P3ID = uint8(k);
                                    P3Range = Range(k);
                                end
                            end
                        end
                    end
                else  % After lost Target  Replaced  1\2\3 Cnt ！
                    if (Range(k)<(TarLimDx+temp))
                        if (spw(k)>=0.8)||((wCutIn(k)>0.7)&&(spw(k)>=0.4))
                            if Range(k)<P0Range
                                P0ID = uint8(k);
                                P0Range = Range(k);
                            end
                        else
                            if spwLeft(k)>0.2
                                if Range(k)<P2Range
                                    P2ID = uint8(k);
                                    P2Range = Range(k);
                                end
                            end
                            if spwLeft(k)>0.2
                                if Range(k)<P3Range
                                    P3ID = uint8(k);
                                    P3Range = Range(k);
                                end
                            end
                        end
                    end
                end %  After lost Target Replaced  //end 
                for i=1:15
                    if (i~=k)&&(Valid(i)==1)&&...
                            (((vRef<=15.83)&&((MoveSts(i)==1)||(MoveSts(i)==2)||(MoveSts(i)==3)))||...
                            ((vRef>15.83)&&((MoveSts(i)==2)||(MoveSts(i)==3))))
                        if (Classfication(i)==1)||(Classfication(i)==2)||(Classfication(i)==3)||(Classfication(i)==9)
                            if ((Range(i)<=TarLimS0Dx)&&(MoveSts(i)==1))||((Range(i)<=TarLimDx)&&((MoveSts(i)==2)||(MoveSts(i)==3)))
                                if (plaus(i)>=0.4)||((wCutIn(i)>0.7)&&(spw(i)>=0.8))||((spw(i)>0.95)&&(Range(i)<1.5*vRef))
                                    if Range(i)<P0Range
                                        P0ID = uint8(i);
                                        P0Range = Range(i);
                                    end
                                else
                                    if spwLeft(i)>0.2
                                        if Range(i)<P2Range
                                            P2ID = uint8(i);
                                            P2Range = Range(i);
                                        end
                                    end
                                    if spwRight(i)>0.2
                                        if Range(i)<P3Range
                                            P3ID = uint8(i);
                                            P3Range = Range(i);
                                        end
                                    end
                                end
                            end
                        end
                    end
                end
            end
        else
            temp = interpolate(single(5),single(10),single(30),single(20),vRef);
            if (ReRange<(TarLimDx+temp))&&(tTargetLost<0.6)
                if (ReDyc<(DycOffset + dyLaneWidth))&&(ReDyc>(-dyLaneWidth - DycOffset))
                   P0ID = k;
                   P0Range = ReRange;
                end
            end
            for i=1:15
                if (Valid(i)==1)&&...
                        (((vRef<=15.83)&&((MoveSts(i)==1)||(MoveSts(i)==2)||(MoveSts(i)==3)))||...
                        ((vRef>15.83)&&((MoveSts(i)==2)||(MoveSts(i)==3))))
                    if (Classfication(i)==1)||(Classfication(i)==2)||(Classfication(i)==3)||(Classfication(i)==9)
                        if ((Range(i)<=TarLimS0Dx)&&(MoveSts(i)==1))||((Range(i)<=TarLimDx)&&((MoveSts(i)==2)||(MoveSts(i)==3)))
                            if (plaus(i)>=0.4)||((wCutIn(i)>0.7)&&(spw(i)>=0.8))||((spw(i)>0.95)&&(Range(i)<1.5*vRef))
                                if Range(i)<P0Range
                                    P0ID = uint8(i);
                                    P0Range = Range(i);
                                end
                            else
                                if spwLeft(i)>0.2
                                    if Range(i)<P2Range
                                        P2ID = uint8(i);
                                        P2Range = Range(i);
                                    end
                                end
                                if spwRight(i)>0.2
                                    if Range(i)<P3Range
                                        P3ID = uint8(i);
                                        P3Range = Range(i);
                                    end
                                end
                            end
                        end
                    end
                end
            end           
        end
    end
end

if (P0ID>0)&&(P0ID<100)
    TargetExist = true;
    P0Range = Range(P0ID);
    P0Vr = Vr(P0ID);
    P0ArG = ArG(P0ID);
    P0Dx = Dx(P0ID);
    P0Dy = Dy(P0ID);
    if wCutIn(P0ID)>0.6
       TargetCutIn_b = true;
    end
    P0Dyc = Dyc(P0ID);
    P0Vyc = Vyc(P0ID);
else
    if P0ID>100
        TargetExist = true;
        P0Range = ReRange;
        P0Vr = ReVx;
        P0ArG = ReArG;
        P0Dx = ReDx;
        P0Dy = ReDy;
        TargetCutIn_b = ReCutIn_b;
        P0Dyc = ReDyc;
        P0Vyc = ReVyc;
    end
end
if P2ID>0
    P2Range = Range(P2ID);
    P2Vr = Vr(P2ID);
    P2ArG = ArG(P2ID);
    P2Dx = Dx(P2ID);
    P2Dy = Dy(P2ID);
end
if P3ID>0
    P3Range = Range(P3ID);
    P3Vr = Vr(P3ID);
    P3ArG = ArG(P3ID);
    P3Dx = Dx(P3ID);
    P3Dy = Dy(P3ID);
end
end

== matlab function Noa_Nofusion_backup/Subsystem2/ACCOSM/HWA_Task100ms1/TimeCalc ==
  data: SameTarget input boolean size=1; TargetID input uint8 size=1; tSameHandleTK1 input single size=1; tSameHandleT output single size=1
function tSameHandleT = TimeCalc(SameTarget,TargetID,tSameHandleTK1)

if TargetID~=0
    if SameTarget==true
        tSameHandleT = min(tSameHandleTK1 + single(0.1),single(1800));
    else
        tSameHandleT = single(0);
    end
else
    tSameHandleT = single(0);
end

== matlab function Noa_Nofusion_backup/Subsystem2/ACCOSM/HWA_Task100ms1/Trajectory/Trajectory/AssignHighPriorityObjects ==
  data: ObjNumber input; TrajNumber input; BufNumber input; SlipDisLim input; ObjPrio input; ObjMatrix input; VxvRef input; ObjCntAlive input; ObjClass input; ObjDxv input; ObjDyv input; TrajUsedK1 input; TrajHistBufferBTrajEndK1 input; ObjTrajNumberK1 input; TrajCurrentIndexK1 input; TrajHistBufferBValidK1 input; TrajHistBufferDxvK1 input; TrajHistBufferDyvK1 input; TrajHistBufferTTimeStampK1 input; TrajHistBufferClassK1 input; TrajUsed output boolean; TrajHistBufferBTrajEnd output boolean; ObjTrajNumber output uint8; TrajCurrentIndex output uint8; TrajHistBufferBValid output boolean; TrajHistBufferDxv output single; TrajHistBufferDyv output single; TrajHistBufferTTimeStamp output single; TrajHistBufferClass output uint8
function [TrajUsed,TrajHistBufferBTrajEnd,ObjTrajNumber,TrajCurrentIndex,TrajHistBufferBValid,...
    TrajHistBufferDxv,TrajHistBufferDyv,...
    TrajHistBufferTTimeStamp,TrajHistBufferClass] = fcn(...
    ObjNumber,TrajNumber,BufNumber,SlipDisLim,ObjPrio,ObjMatrix,VxvRef,ObjCntAlive,ObjClass,ObjDxv,ObjDyv,...
    TrajUsedK1,TrajHistBufferBTrajEndK1,ObjTrajNumberK1,TrajCurrentIndexK1,...
    TrajHistBufferBValidK1,TrajHistBufferDxvK1,TrajHistBufferDyvK1,...
    TrajHistBufferTTimeStampK1,TrajHistBufferClassK1)

[TrajUsed,TrajHistBufferBTrajEnd,ObjTrajNumber,TrajCurrentIndex,TrajHistBufferBValid,...
    TrajHistBufferDxv,TrajHistBufferDyv,...
    TrajHistBufferTTimeStamp,TrajHistBufferClass] = Traj_AssignHighPriorityObjects(...
    ObjNumber,TrajNumber,BufNumber,SlipDisLim,ObjPrio,ObjMatrix,VxvRef,ObjCntAlive,ObjClass,ObjDxv,ObjDyv,...
    TrajUsedK1,TrajHistBufferBTrajEndK1,ObjTrajNumberK1,TrajCurrentIndexK1,...
    TrajHistBufferBValidK1,TrajHistBufferDxvK1,TrajHistBufferDyvK1,...
    TrajHistBufferTTimeStampK1,TrajHistBufferClassK1);
end

== matlab function Noa_Nofusion_backup/Subsystem2/ACCOSM/HWA_Task100ms1/Trajectory/Trajectory/CalcCompensateEgoVehMove ==
  data: BufNumber input; TrajNumber input; tCycle input; dDeltaX input; dDeltaY input; CosOfPsi input; SinOfPsi input; TrajHistBufferBValidK1 input; TrajHistBufferDxvK1 input; TrajHistBufferDyvK1 input; TrajHistBufferBValid output; TrajHistBufferDxv output; TrajHistBufferDyv output; TrajHistBufferTTimeStampK1 input; TrajHistBufferTTimeStamp output
function [TrajHistBufferBValid,TrajHistBufferDxv,TrajHistBufferDyv,...
    TrajHistBufferTTimeStamp] = ...
    Compensate(BufNumber,TrajNumber,tCycle,dDeltaX,dDeltaY,CosOfPsi,SinOfPsi,...
    TrajHistBufferBValidK1,TrajHistBufferDxvK1,TrajHistBufferDyvK1,...
    TrajHistBufferTTimeStampK1)
%#codegen
TrajHistBufferBValid = TrajHistBufferBValidK1;
TrajHistBufferDxv = TrajHistBufferDxvK1;
TrajHistBufferDyv = TrajHistBufferDyvK1;
TrajHistBufferTTimeStamp = TrajHistBufferTTimeStampK1;

for i=1:TrajNumber
    for j=1:BufNumber
        if TrajHistBufferBValid(i,j)==true
            t_dx = TrajHistBufferDxv(i,j)-dDeltaX;
            t_dy = TrajHistBufferDyv(i,j)-dDeltaY;
            t_dxTmp = t_dx*CosOfPsi+t_dy*SinOfPsi;
            t_dyTmp = -t_dx*SinOfPsi+t_dy*CosOfPsi;
            if (t_dxTmp>-255)&&(t_dxTmp<255)&&(t_dyTmp>-255)&&(t_dyTmp<255)
                TrajHistBufferDxv(i,j) = t_dxTmp;
                TrajHistBufferDyv(i,j) = t_dyTmp;
            else
                TrajHistBufferBValid(i,j) = false;
            end
            
            TrajHistBufferTTimeStamp(i,j) = min(TrajHistBufferTTimeStamp(i,j)+tCycle,32);
            
            if TrajHistBufferDxv(i,j)<-1
                TrajHistBufferBValid(i,j) = false;
            end
        end
    end
end
